simulink model "myss_p1_ej2"  (R2022b)
settings: Solver=VariableStepAuto  StartTime=0.0  StopTime=10.0  RelTol=1e-3
settings Model: Creator=adrub  LastModifiedBy=adrub

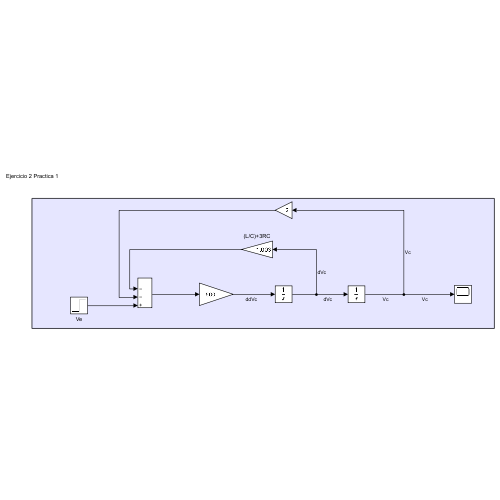
[thumbnail: Simulink's stored preview of the top-level diagram]
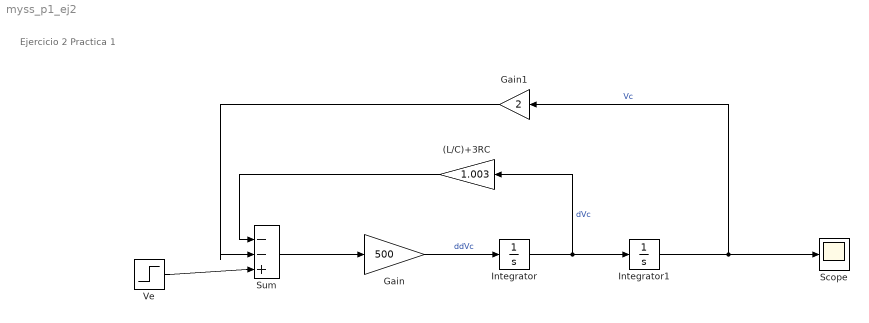
== system myss_p1_ej2 ==
  note: Ejercicio 2 Practica 1
  (L/C)+3RC : Gain  Gain=1.003
  Gain : Gain  Gain=500
  Gain1 : Gain  Gain=2
  Integrator : Integrator
  Integrator1 : Integrator
  Scope : Scope
  Sum : Sum  Inputs=|--+
  Ve : Step  Before=1  SampleTime=0
  wires:
  Ve/1 -> Sum/3
  Sum/1 -> Gain/1
  Integrator/1 -> (L/C)+3RC/1, Integrator1/1  "dVc"
  Gain/1 -> Integrator/1  "ddVc"
  Integrator1/1 -> Gain1/1, Scope/1  "Vc"
  Gain1/1 -> Sum/2
  (L/C)+3RC/1 -> Sum/1
